simulink model "mulacc"  (R2024b)
settings: Solver=VariableStepAuto  StartTime=0.0  StopTime=inf  RelTol=1e-3
libraries: slrealtimeiplib x3, simulink x2, slrealtimeutilitieslib x2
settings Model: Creator=shaniaki  LastModifiedBy=marmar
settings RTWCC: GPUComputeCapability=3.5

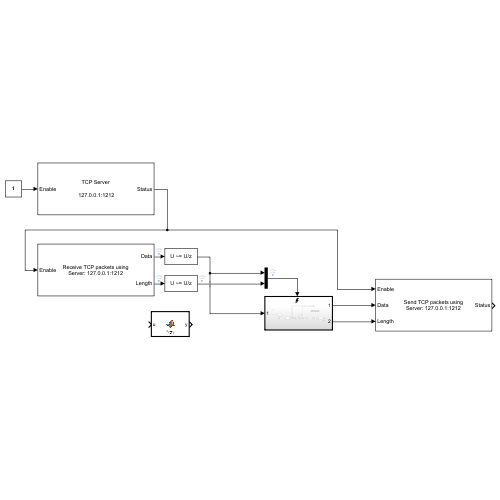
[thumbnail: Simulink's stored preview of the top-level diagram]
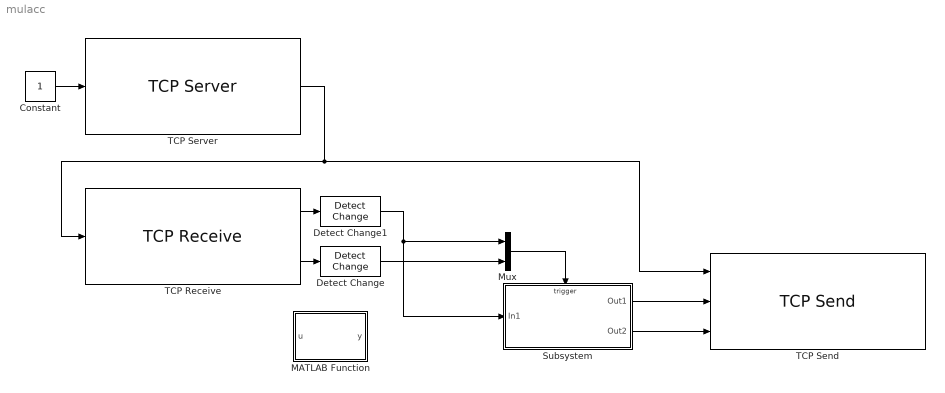
== system mulacc ==
  Constant : Constant
  Detect Change : simulink/Logic and Bit Operations/Detect Change  vinit=0  OutDataTypeStr=boolean
  Detect Change1 : simulink/Logic and Bit Operations/Detect Change  vinit=0  OutDataTypeStr=boolean
  MATLAB Function : MATLAB Function  TreatAsAtomicUnit=on
  Mux : Mux  Inputs=2
  Subsystem : Subsystem
  TCP Receive : slrealtimeiplib/TCP Receive  socketAddPortVal=Server: 127.0.0.1:1212  rcvWidth=16  sampleTime=-1
  TCP Send : slrealtimeiplib/TCP Send  socketAddPortVal=Server: 127.0.0.1:1212  sampleTime=-1
  TCP Server : slrealtimeiplib/TCP Server  Priority=-1  useHostTargetConn=off  serverAddress=127.0.0.1  serverPort=1212
  wires:
  TCP Server/1 -> TCP Receive/1, TCP Send/1
  Constant/1 -> TCP Server/1
  TCP Receive/2 -> Detect Change/1
  TCP Receive/1 -> Detect Change1/1
  Subsystem/1(Out1) -> TCP Send/2
  Subsystem/2(Out2) -> TCP Send/3
  Detect Change/1 -> Mux/2
  Detect Change1/1 -> Subsystem/1(In1), Mux/1
  Mux/1 -> Subsystem/Trigger

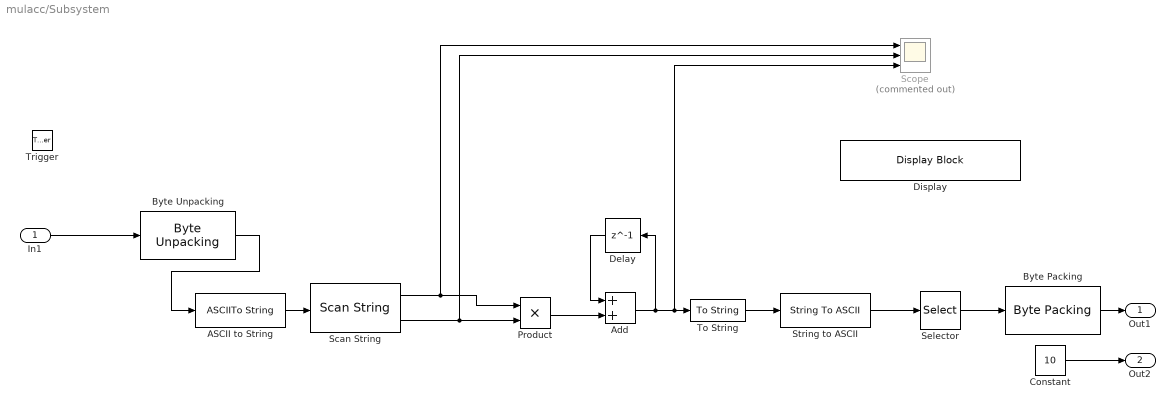
== system mulacc/Subsystem ==
  In1 : Inport
  Trigger : TriggerPort  VariantControl=(inherit)  PortDimensions=1
  ASCII to String : ASCIIToString
  Add : Sum
  Byte Packing : slrealtimeutilitieslib/Byte Packing  MaskPackedDataType=uint8  MaskUnpackedDataTypes={'uint8'}  MaskAlignment=1
  Byte Unpacking : slrealtimeutilitieslib/Byte Unpacking  MaskUnpackedDataTypes={'uint8'}  MaskUnpackedDataSizes={[16]}  MaskAlignment=1
  Constant : Constant  Value=10
  Delay : Delay  DelayLength=1
  Display : DisplayBlock  LabelPosition=Hide  Format=Custom  Transparency=1  FormatString=%s
  Product : Product
  Scan String : ScanString  Format="\"%d %d\""
  Scope : Scope  Commented=on  NumInputPorts=3
  Selector : Selector  InputPortWidth=31  IndexOptions=Index vector (dialog)  Indices=[1 10]  OutputSizes=1
  String to ASCII : StringToASCII
  To String : ToString
  Out1 : Outport
  Out2 : Outport  Port=2
  wires:
  Delay/1 -> Add/1
  Product/1 -> Add/2
  ASCII to String/1 -> Scan String/1
  Byte Unpacking/1 -> ASCII to String/1
  Scan String/1 -> Scope/1, Product/1
  Scan String/2 -> Scope/2, Product/2
  Add/1 -> Scope/3, To String/1, Delay/1
  To String/1 -> String to ASCII/1
  In1/1 -> Byte Unpacking/1
  String to ASCII/1 -> Selector/1
  Byte Packing/1 -> Out1/1
  Selector/1 -> Byte Packing/1
  Constant/1 -> Out2/1

== matlab function mulacc/MATLAB Function ==
  data: u input; y output
function y = fcn(u)

y = u;
